simulink model "Lab7_4"  (R2023a)
settings: Solver=FixedStepAuto  StartTime=0.0  StopTime=3.0  FixedStep=0.0001  RelTol=1e-3
undefined symbols (not defined in the file): A, B, C, D, x_0
settings Model: Creator=Дети  LastModifiedBy=user
settings OptimizationCC: ReuseModelBlockBuffer=off

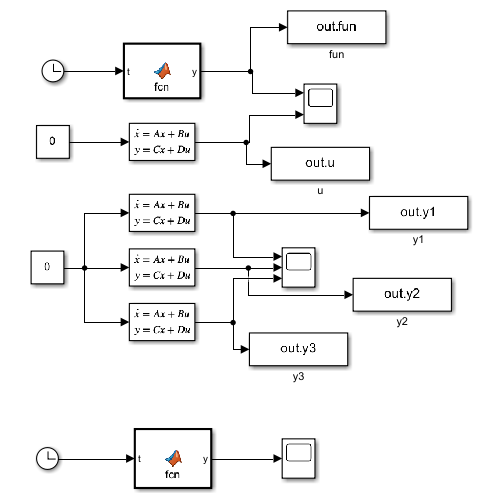
[thumbnail: Simulink's stored preview of the top-level diagram]
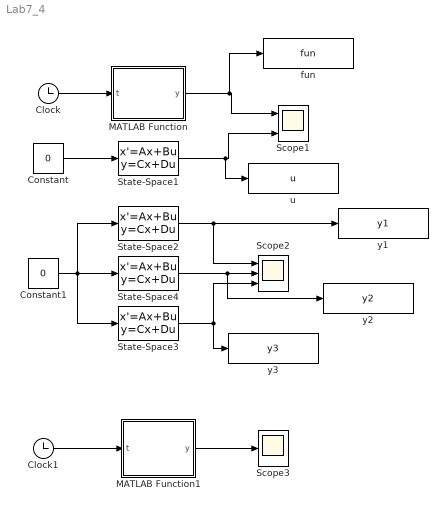
== system Lab7_4 ==
  Clock : Clock
  Clock1 : Clock
  Constant : Constant  Value=0
  Constant1 : Constant  Value=0
  MATLAB Function : MATLAB Function  TreatAsAtomicUnit=on
  MATLAB Function1 : MATLAB Function  TreatAsAtomicUnit=on
  Scope1 : Scope  NumInputPorts=2
  Scope2 : Scope  NumInputPorts=3
  Scope3 : Scope
  State-Space1 : StateSpace  A=A  B=B  C=C  D=D  InitialCondition=[-4.3988; 0.6012; 1.3988]  ParameterTunability=Unconstrained
  State-Space2 : StateSpace  A=A  B=B  C=[1 0 0]  D=D  InitialCondition=[-4.3988; 0.6012; 1.3988]  ParameterTunability=Unconstrained
  State-Space3 : StateSpace  A=A  B=B  C=[0 0 1]  D=D  InitialCondition=[-4.3988; 0.6012; 1.3988]
  State-Space4 : StateSpace  A=A  B=B  C=[0 1 0]  D=D  InitialCondition=[-4.3988; 0.6012; 1.3988]
  fun : ToWorkspace  VariableName=fun  SaveFormat=Timeseries  SampleTime=-1
  u : ToWorkspace  VariableName=u  SaveFormat=Timeseries  SampleTime=-1
  y1 : ToWorkspace  VariableName=y1  SaveFormat=Timeseries  SampleTime=-1
  y2 : ToWorkspace  VariableName=y2  SaveFormat=Timeseries  SampleTime=-1
  y3 : ToWorkspace  VariableName=y3  SaveFormat=Timeseries  SampleTime=-1
  wires:
  Clock/1 -> MATLAB Function/1(t)
  State-Space1/1 -> u/1, Scope1/2
  Constant/1 -> State-Space1/1
  MATLAB Function/1(y) -> fun/1, Scope1/1
  State-Space2/1 -> y1/1, Scope2/1
  State-Space4/1 -> y2/1, Scope2/2
  State-Space3/1 -> y3/1, Scope2/3
  Constant1/1 -> State-Space3/1, State-Space2/1, State-Space4/1
  Clock1/1 -> MATLAB Function1/1(t)
  MATLAB Function1/1(y) -> Scope3/1

== matlab function Lab7_4/MATLAB Function1 ==
  data: t input; y output; A parameter; x_0 parameter
function y = fcn(t, A, x_0)
y = expm(A*t)*x_0;

== matlab function Lab7_4/MATLAB Function ==
  data: t input; y output
function y = fcn(t)
y = (-3)*exp(-3*t)*cos(2*t) - 2*exp(-3*t)*sin(2*t);
